simulink model "ExtendedLQR"  (R2020b)
settings: Solver=ode45  StartTime=0.0  StopTime=3  RelTol=1e-4
values from neighbouring files (symbols this model uses):
  degs2rpm = 60/360    (= 0.166666666667)    [load_params_inertial_case.m]
  rads2rpm = 60/2/pi    (= 9.54929658551)    [load_params_inertial_case.m]
  rpm2rads = 2*pi/60    (= 0.10471975512)    [load_params_inertial_case.m]
undefined symbols (not defined in the file or in its folder): daq, drv, extended_bryson_lqr, extended_lqr, gbox, mld, mot, sens, state_space
settings Model: Creator=Utente  LastModifiedBy=Utente
settings SolverCC: ZeroCrossAlgorithm=Adaptive
settings DataIOCC: ReturnWorkspaceOutputs=off
settings DebuggingCC: IgnoredZcDiagnostic=none

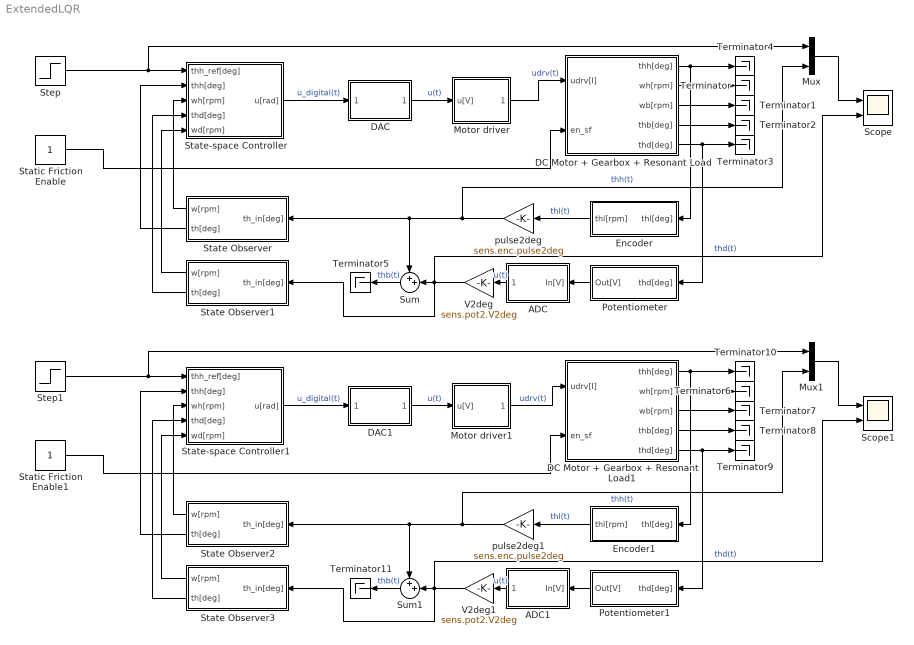
== system ExtendedLQR ==
  ADC : Subsystem
  ADC1 : Subsystem
  DAC : Subsystem
  DAC1 : Subsystem
  DC Motor + Gearbox + Resonant Load : Subsystem
  DC Motor + Gearbox + Resonant Load1 : Subsystem
  Encoder : Subsystem
  Encoder1 : Subsystem
  Motor driver : Subsystem
  Motor driver1 : Subsystem
  Mux : Mux  Inputs=2
  Mux1 : Mux  Inputs=2
  Potentiometer : Subsystem
  Potentiometer1 : Subsystem
  Scope : Scope  NumInputPorts=2
  Scope1 : Scope  NumInputPorts=2
  State Observer : Subsystem
  State Observer1 : Subsystem
  State Observer2 : Subsystem
  State Observer3 : Subsystem
  State-space Controller : Subsystem
  State-space Controller1 : Subsystem
  Static Friction Enable : Constant
  Static Friction Enable1 : Constant
  Step : Step  Time=0  After=50  SampleTime=0
  Step1 : Step  Time=0  After=50  SampleTime=0
  Sum : Sum  Inputs=++|
  Sum1 : Sum  Inputs=++|
  Terminator{,1..11} (12 alike) : Terminator
  V2deg : Gain  Gain=sens.pot2.V2deg
  V2deg1 : Gain  Gain=sens.pot2.V2deg
  pulse2deg : Gain  Gain=sens.enc.pulse2deg
  pulse2deg1 : Gain  Gain=sens.enc.pulse2deg
  wires:
  DC Motor + Gearbox + Resonant Load/5(thd[deg]) -> Terminator3/1, Potentiometer/1(thd[deg])
  DC Motor + Gearbox + Resonant Load/1(thh[deg]) -> Terminator4/1, Encoder/1(thl[deg])
  DC Motor + Gearbox + Resonant Load/2(wh[rpm]) -> Terminator/1
  DC Motor + Gearbox + Resonant Load/3(wb[rpm]) -> Terminator1/1
  DC Motor + Gearbox + Resonant Load/4(thb[deg]) -> Terminator2/1
  Encoder/1(thl[rpm]) -> pulse2deg/1  "thl(t)"
  V2deg/1 -> State Observer1/1(th_in[deg]), Scope/2, Sum/2  "thd(t)"
  pulse2deg/1 -> Mux/2, State Observer/1(th_in[deg]), Sum/1  "thh(t)"
  Motor driver/1(udrv[I]) -> DC Motor + Gearbox + Resonant Load/1(udrv[I])  "udrv(t)"
  DAC/1(Out[V]) -> Motor driver/1(u[V])  "u(t)"
  ADC/1(Out[V]) -> V2deg/1  "u(t)"
  Potentiometer/1(Out[V]) -> ADC/1(In[V])
  State-space Controller/1(u[rad]) -> DAC/1(In[rad])  "u_digital(t)"
  Step/1 -> State-space Controller/1(thh_ref[deg]), Mux/1
  Mux/1 -> Scope/1
  State Observer/1(w[rpm]) -> State-space Controller/3(wh[rpm])
  State Observer/2(th[deg]) -> State-space Controller/2(thh[deg])
  State Observer1/1(w[rpm]) -> State-space Controller/5(wd[rpm])
  State Observer1/2(th[deg]) -> State-space Controller/4(thd[deg])
  Sum/1 -> Terminator5/1  "thb(t)"
  Static Friction Enable/1 -> DC Motor + Gearbox + Resonant Load/2(en_sf)
  Step1/1 -> State-space Controller1/1(thh_ref[deg]), Mux1/1
  Static Friction Enable1/1 -> DC Motor + Gearbox + Resonant Load1/2(en_sf)
  State Observer2/2(th[deg]) -> State-space Controller1/2(thh[deg])
  Potentiometer1/1(Out[V]) -> ADC1/1(In[V])
  State Observer3/1(w[rpm]) -> State-space Controller1/5(wd[rpm])
  State Observer3/2(th[deg]) -> State-space Controller1/4(thd[deg])
  Encoder1/1(thl[rpm]) -> pulse2deg1/1  "thl(t)"
  V2deg1/1 -> State Observer3/1(th_in[deg]), Scope1/2, Sum1/2  "thd(t)"
  DAC1/1(Out[V]) -> Motor driver1/1(u[V])  "u(t)"
  State-space Controller1/1(u[rad]) -> DAC1/1(In[rad])  "u_digital(t)"
  Mux1/1 -> Scope1/1
  State Observer2/1(w[rpm]) -> State-space Controller1/3(wh[rpm])
  DC Motor + Gearbox + Resonant Load1/3(wb[rpm]) -> Terminator7/1
  ADC1/1(Out[V]) -> V2deg1/1  "u(t)"
  DC Motor + Gearbox + Resonant Load1/1(thh[deg]) -> Terminator10/1, Encoder1/1(thl[deg])
  Sum1/1 -> Terminator11/1  "thb(t)"
  Motor driver1/1(udrv[I]) -> DC Motor + Gearbox + Resonant Load1/1(udrv[I])  "udrv(t)"
  DC Motor + Gearbox + Resonant Load1/4(thb[deg]) -> Terminator8/1
  pulse2deg1/1 -> Mux1/2, State Observer2/1(th_in[deg]), Sum1/1  "thh(t)"
  DC Motor + Gearbox + Resonant Load1/2(wh[rpm]) -> Terminator6/1
  DC Motor + Gearbox + Resonant Load1/5(thd[deg]) -> Terminator9/1, Potentiometer1/1(thd[deg])

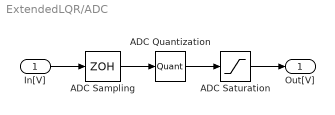
== system ExtendedLQR/ADC ==
  In[V] : Inport
  ADC Quantization : Quantizer  QuantizationInterval=daq.adc.q
  ADC Sampling : ZeroOrderHold  SampleTime=daq.adc.T_s
  ADC Saturation : Saturate  UpperLimit=daq.adc.vdd  LowerLimit=daq.adc.vss
  Out[V] : Outport
  wires:
  ADC Quantization/1 -> ADC Saturation/1
  ADC Sampling/1 -> ADC Quantization/1
  ADC Saturation/1 -> Out[V]/1
  In[V]/1 -> ADC Sampling/1

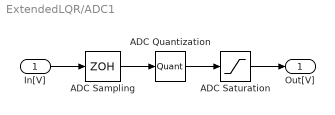
== system ExtendedLQR/ADC1 ==
  In[V] : Inport
  ADC Quantization : Quantizer  QuantizationInterval=daq.adc.q
  ADC Sampling : ZeroOrderHold  SampleTime=daq.adc.T_s
  ADC Saturation : Saturate  UpperLimit=daq.adc.vdd  LowerLimit=daq.adc.vss
  Out[V] : Outport
  wires:
  ADC Quantization/1 -> ADC Saturation/1
  ADC Sampling/1 -> ADC Quantization/1
  ADC Saturation/1 -> Out[V]/1
  In[V]/1 -> ADC Sampling/1

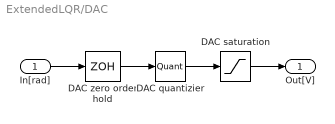
== system ExtendedLQR/DAC ==
  In[rad] : Inport
  DAC quantizier : Quantizer  QuantizationInterval=daq.dac.q
  DAC saturation : Saturate  UpperLimit=daq.dac.vdd  LowerLimit=daq.dac.vss
  DAC zero order hold : ZeroOrderHold  SampleTime=daq.dac.T_s
  Out[V] : Outport
  wires:
  DAC quantizier/1 -> DAC saturation/1
  DAC zero order hold/1 -> DAC quantizier/1
  DAC saturation/1 -> Out[V]/1
  In[rad]/1 -> DAC zero order hold/1

== system ExtendedLQR/DAC1 ==
  In[rad] : Inport
  DAC quantizier : Quantizer  QuantizationInterval=daq.dac.q
  DAC saturation : Saturate  UpperLimit=daq.dac.vdd  LowerLimit=daq.dac.vss
  DAC zero order hold : ZeroOrderHold  SampleTime=daq.dac.T_s
  Out[V] : Outport
  wires:
  DAC quantizier/1 -> DAC saturation/1
  DAC zero order hold/1 -> DAC quantizier/1
  DAC saturation/1 -> Out[V]/1
  In[rad]/1 -> DAC zero order hold/1

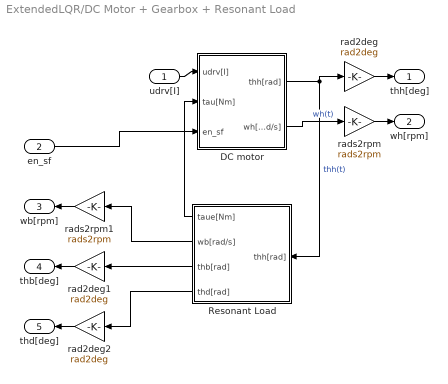
== system ExtendedLQR/DC Motor + Gearbox + Resonant Load ==
  udrv[I] : Inport
  en_sf : Inport  Port=2
  DC motor : Subsystem
  Resonant Load : Subsystem
  rad2deg : Gain  Gain=rad2deg
  rad2deg1 : Gain  Gain=rad2deg
  rad2deg2 : Gain  Gain=rad2deg
  rads2rpm : Gain  Gain=rads2rpm
  rads2rpm1 : Gain  Gain=rads2rpm
  thh[deg] : Outport
  wh[rpm] : Outport  Port=2
  wb[rpm] : Outport  Port=3
  thb[deg] : Outport  Port=4
  thd[deg] : Outport  Port=5
  wires:
  rad2deg2/1 -> thd[deg]/1
  rad2deg1/1 -> thb[deg]/1
  DC motor/1(thh[rad]) -> rad2deg/1, Resonant Load/1(thh[rad])  "thh(t)"
  Resonant Load/2(wb[rad/s]) -> rads2rpm1/1
  Resonant Load/4(thd[rad]) -> rad2deg2/1
  Resonant Load/3(thb[rad]) -> rad2deg1/1
  DC motor/2(wh[rad/s]) -> rads2rpm/1  "wh(t)"
  udrv[I]/1 -> DC motor/1(udrv[I])
  rad2deg/1 -> thh[deg]/1
  rads2rpm/1 -> wh[rpm]/1
  rads2rpm1/1 -> wb[rpm]/1
  Resonant Load/1(taue[Nm]) -> DC motor/2(tau[Nm])
  en_sf/1 -> DC motor/3(en_sf)

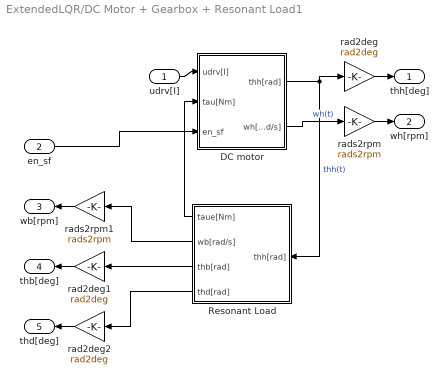
== system ExtendedLQR/DC Motor + Gearbox + Resonant Load1 ==
  udrv[I] : Inport
  en_sf : Inport  Port=2
  DC motor : Subsystem
  Resonant Load : Subsystem
  rad2deg : Gain  Gain=rad2deg
  rad2deg1 : Gain  Gain=rad2deg
  rad2deg2 : Gain  Gain=rad2deg
  rads2rpm : Gain  Gain=rads2rpm
  rads2rpm1 : Gain  Gain=rads2rpm
  thh[deg] : Outport
  wh[rpm] : Outport  Port=2
  wb[rpm] : Outport  Port=3
  thb[deg] : Outport  Port=4
  thd[deg] : Outport  Port=5
  wires:
  rad2deg2/1 -> thd[deg]/1
  rad2deg1/1 -> thb[deg]/1
  DC motor/1(thh[rad]) -> rad2deg/1, Resonant Load/1(thh[rad])  "thh(t)"
  Resonant Load/2(wb[rad/s]) -> rads2rpm1/1
  Resonant Load/4(thd[rad]) -> rad2deg2/1
  Resonant Load/3(thb[rad]) -> rad2deg1/1
  DC motor/2(wh[rad/s]) -> rads2rpm/1  "wh(t)"
  udrv[I]/1 -> DC motor/1(udrv[I])
  rad2deg/1 -> thh[deg]/1
  rads2rpm/1 -> wh[rpm]/1
  rads2rpm1/1 -> wb[rpm]/1
  Resonant Load/1(taue[Nm]) -> DC motor/2(tau[Nm])
  en_sf/1 -> DC motor/3(en_sf)

== system ExtendedLQR/Encoder ==
  thl[deg] : Inport
  Encoder quantization : Quantizer  QuantizationInterval=sens.enc.q
  Encoder sampling : ZeroOrderHold  SampleTime=sens.enc.T_s
  deg2pulse : Gain  Gain=sens.enc.deg2pulse
  thl[rpm] : Outport
  wires:
  Encoder quantization/1 -> deg2pulse/1
  deg2pulse/1 -> thl[rpm]/1
  Encoder sampling/1 -> Encoder quantization/1
  thl[deg]/1 -> Encoder sampling/1

== system ExtendedLQR/Encoder1 ==
  thl[deg] : Inport
  Encoder quantization : Quantizer  QuantizationInterval=sens.enc.q
  Encoder sampling : ZeroOrderHold  SampleTime=sens.enc.T_s
  deg2pulse : Gain  Gain=sens.enc.deg2pulse
  thl[rpm] : Outport
  wires:
  Encoder quantization/1 -> deg2pulse/1
  deg2pulse/1 -> thl[rpm]/1
  Encoder sampling/1 -> Encoder quantization/1
  thl[deg]/1 -> Encoder sampling/1

== system ExtendedLQR/Motor driver ==
  u[V] : Inport
  Driver dynamics : TransferFcn  Numerator=[drv.dcgain]  Denominator=[drv.Tc 1]
  Driver saturation : Saturate  UpperLimit=drv.vp  LowerLimit=drv.vm
  udrv[I] : Outport
  wires:
  Driver saturation/1 -> udrv[I]/1
  Driver dynamics/1 -> Driver saturation/1
  u[V]/1 -> Driver dynamics/1

== system ExtendedLQR/Motor driver1 ==
  u[V] : Inport
  Driver dynamics : TransferFcn  Numerator=[drv.dcgain]  Denominator=[drv.Tc 1]
  Driver saturation : Saturate  UpperLimit=drv.vp  LowerLimit=drv.vm
  udrv[I] : Outport
  wires:
  Driver saturation/1 -> udrv[I]/1
  Driver dynamics/1 -> Driver saturation/1
  u[V]/1 -> Driver dynamics/1

== system ExtendedLQR/Potentiometer ==
  thd[deg] : Inport
  Sensor Output Noise [V] : RandomNumber  Variance=sens.pot2.noise.var  SampleTime=0.1
  Sum : Sum  Inputs=|++
  deg2V : Gain  Gain=sens.pot2.deg2V
  Out[V] : Outport
  wires:
  thd[deg]/1 -> deg2V/1
  Sensor Output Noise [V]/1 -> Sum/2
  deg2V/1 -> Sum/1
  Sum/1 -> Out[V]/1

== system ExtendedLQR/Potentiometer1 ==
  thd[deg] : Inport
  Sensor Output Noise [V] : RandomNumber  Variance=sens.pot2.noise.var  SampleTime=0.1
  Sum : Sum  Inputs=|++
  deg2V : Gain  Gain=sens.pot2.deg2V
  Out[V] : Outport
  wires:
  thd[deg]/1 -> deg2V/1
  Sensor Output Noise [V]/1 -> Sum/2
  deg2V/1 -> Sum/1
  Sum/1 -> Out[V]/1

== system ExtendedLQR/State Observer ==
  th_in[deg] : Inport
  Derivator : TransferFcn  Numerator=[state_space.obs.wc^2 0]  Denominator=[1 2*state_space.obs.delta*state_space.obs.wc state_space.obs.wc^2]
  degs2rpm : Gain  Gain=degs2rpm
  w[rpm] : Outport
  th[deg] : Outport  Port=2
  wires:
  Derivator/1 -> degs2rpm/1
  th_in[deg]/1 -> th[deg]/1, Derivator/1
  degs2rpm/1 -> w[rpm]/1

== system ExtendedLQR/State Observer1 ==
  th_in[deg] : Inport
  Transfer Fcn : TransferFcn  Numerator=[state_space.obs.wc^2 0]  Denominator=[1 2*state_space.obs.delta*state_space.obs.wc state_space.obs.wc^2]
  degs2rpm : Gain  Gain=degs2rpm
  w[rpm] : Outport
  th[deg] : Outport  Port=2
  wires:
  Transfer Fcn/1 -> degs2rpm/1
  th_in[deg]/1 -> th[deg]/1, Transfer Fcn/1
  degs2rpm/1 -> w[rpm]/1

== system ExtendedLQR/State Observer2 ==
  th_in[deg] : Inport
  Derivator : TransferFcn  Numerator=[state_space.obs.wc^2 0]  Denominator=[1 2*state_space.obs.delta*state_space.obs.wc state_space.obs.wc^2]
  degs2rpm : Gain  Gain=degs2rpm
  w[rpm] : Outport
  th[deg] : Outport  Port=2
  wires:
  Derivator/1 -> degs2rpm/1
  th_in[deg]/1 -> th[deg]/1, Derivator/1
  degs2rpm/1 -> w[rpm]/1

== system ExtendedLQR/State Observer3 ==
  th_in[deg] : Inport
  Transfer Fcn : TransferFcn  Numerator=[state_space.obs.wc^2 0]  Denominator=[1 2*state_space.obs.delta*state_space.obs.wc state_space.obs.wc^2]
  degs2rpm : Gain  Gain=degs2rpm
  w[rpm] : Outport
  th[deg] : Outport  Port=2
  wires:
  Transfer Fcn/1 -> degs2rpm/1
  th_in[deg]/1 -> th[deg]/1, Transfer Fcn/1
  degs2rpm/1 -> w[rpm]/1

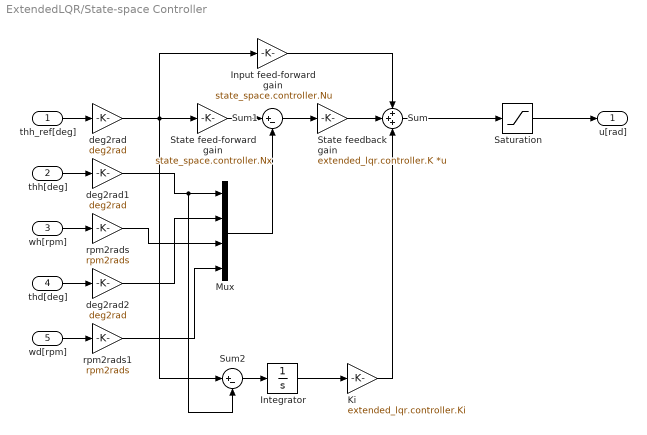
== system ExtendedLQR/State-space Controller ==
  thh_ref[deg] : Inport
  thh[deg] : Inport  Port=2
  wh[rpm] : Inport  Port=3
  thd[deg] : Inport  Port=4
  wd[rpm] : Inport  Port=5
  Input feed-forward gain : Gain  Gain=state_space.controller.Nu
  Integrator : Integrator
  Ki : Gain  Gain=extended_lqr.controller.Ki
  Mux : Mux
  Saturation : Saturate  UpperLimit=daq.dac.vdd  LowerLimit=daq.dac.vss
  State feed-forward gain : Gain  Gain=state_space.controller.Nx
  State feedback gain : Gain  Gain=extended_lqr.controller.K  Multiplication=Matrix(K*u)
  Sum : Sum  Inputs=+++
  Sum1 : Sum  Inputs=|+-
  Sum2 : Sum  Inputs=|+-
  deg2rad : Gain  Gain=deg2rad
  deg2rad1 : Gain  Gain=deg2rad
  deg2rad2 : Gain  Gain=deg2rad
  rpm2rads : Gain  Gain=rpm2rads
  rpm2rads1 : Gain  Gain=rpm2rads
  u[rad] : Outport
  wires:
  Sum1/1 -> State feedback gain/1
  Mux/1 -> Sum1/2
  thh_ref[deg]/1 -> deg2rad/1
  deg2rad/1 -> Sum2/1, Input feed-forward gain/1, State feed-forward gain/1
  State feed-forward gain/1 -> Sum1/1
  Input feed-forward gain/1 -> Sum/1
  Saturation/1 -> u[rad]/1
  wh[rpm]/1 -> rpm2rads/1
  thh[deg]/1 -> deg2rad1/1
  State feedback gain/1 -> Sum/2
  Sum/1 -> Saturation/1
  thd[deg]/1 -> deg2rad2/1
  wd[rpm]/1 -> rpm2rads1/1
  deg2rad1/1 -> Sum2/2, Mux/1
  deg2rad2/1 -> Mux/2
  rpm2rads/1 -> Mux/3
  rpm2rads1/1 -> Mux/4
  Integrator/1 -> Ki/1
  Sum2/1 -> Integrator/1
  Ki/1 -> Sum/3

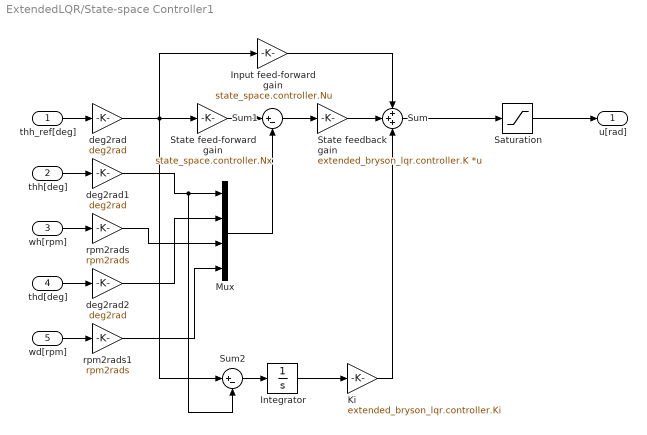
== system ExtendedLQR/State-space Controller1 ==
  thh_ref[deg] : Inport
  thh[deg] : Inport  Port=2
  wh[rpm] : Inport  Port=3
  thd[deg] : Inport  Port=4
  wd[rpm] : Inport  Port=5
  Input feed-forward gain : Gain  Gain=state_space.controller.Nu
  Integrator : Integrator
  Ki : Gain  Gain=extended_bryson_lqr.controller.Ki
  Mux : Mux
  Saturation : Saturate  UpperLimit=daq.dac.vdd  LowerLimit=daq.dac.vss
  State feed-forward gain : Gain  Gain=state_space.controller.Nx
  State feedback gain : Gain  Gain=extended_bryson_lqr.controller.K  Multiplication=Matrix(K*u)
  Sum : Sum  Inputs=+++
  Sum1 : Sum  Inputs=|+-
  Sum2 : Sum  Inputs=|+-
  deg2rad : Gain  Gain=deg2rad
  deg2rad1 : Gain  Gain=deg2rad
  deg2rad2 : Gain  Gain=deg2rad
  rpm2rads : Gain  Gain=rpm2rads
  rpm2rads1 : Gain  Gain=rpm2rads
  u[rad] : Outport
  wires:
  Sum1/1 -> State feedback gain/1
  Mux/1 -> Sum1/2
  thh_ref[deg]/1 -> deg2rad/1
  deg2rad/1 -> Sum2/1, Input feed-forward gain/1, State feed-forward gain/1
  State feed-forward gain/1 -> Sum1/1
  Input feed-forward gain/1 -> Sum/1
  Saturation/1 -> u[rad]/1
  wh[rpm]/1 -> rpm2rads/1
  thh[deg]/1 -> deg2rad1/1
  State feedback gain/1 -> Sum/2
  Sum/1 -> Saturation/1
  thd[deg]/1 -> deg2rad2/1
  wd[rpm]/1 -> rpm2rads1/1
  deg2rad1/1 -> Sum2/2, Mux/1
  deg2rad2/1 -> Mux/2
  rpm2rads/1 -> Mux/3
  rpm2rads1/1 -> Mux/4
  Integrator/1 -> Ki/1
  Sum2/1 -> Integrator/1
  Ki/1 -> Sum/3

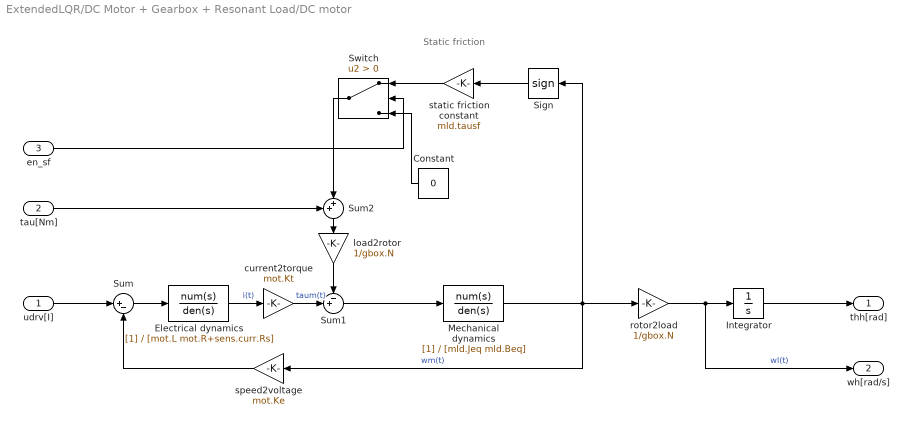
== system ExtendedLQR/DC Motor + Gearbox + Resonant Load/DC motor ==
  note: Static friction
  udrv[I] : Inport  Unit=V
  tau[Nm] : Inport  Port=2  Unit=V
  en_sf : Inport  Port=3  Unit=V
  Constant : Constant  Value=0
  Electrical dynamics : TransferFcn  Denominator=[mot.L mot.R+sens.curr.Rs]
  Integrator : Integrator
  Mechanical dynamics : TransferFcn  Denominator=[mld.Jeq mld.Beq]
  Sign : Signum  ZeroCross=off
  Sum : Sum  Inputs=|+-
  Sum1 : Sum  Inputs=-+|
  Sum2 : Sum  Inputs=++|
  Switch : Switch  Criteria=u2 > Threshold
  current2torque : Gain  Gain=mot.Kt
  load2rotor : Gain  Gain=1/gbox.N
  rotor2load : Gain  Gain=1/gbox.N
  speed2voltage : Gain  Gain=mot.Ke
  static friction constant : Gain  Gain=mld.tausf
  thh[rad] : Outport  Unit=deg
  wh[rad/s] : Outport  Port=2  Unit=rpm
  wires:
  load2rotor/1 -> Sum1/1
  Mechanical dynamics/1 -> Sign/1, rotor2load/1, speed2voltage/1  "wm(t)"
  Sign/1 -> static friction constant/1
  current2torque/1 -> Sum1/2  "taum(t)"
  Sum1/1 -> Mechanical dynamics/1
  speed2voltage/1 -> Sum/2
  rotor2load/1 -> wh[rad/s]/1, Integrator/1  "wl(t)"
  Electrical dynamics/1 -> current2torque/1  "i(t)"
  Sum/1 -> Electrical dynamics/1
  Integrator/1 -> thh[rad]/1
  udrv[I]/1 -> Sum/1
  Sum2/1 -> load2rotor/1
  tau[Nm]/1 -> Sum2/1
  static friction constant/1 -> Switch/1
  Switch/1 -> Sum2/2
  en_sf/1 -> Switch/2
  Constant/1 -> Switch/3

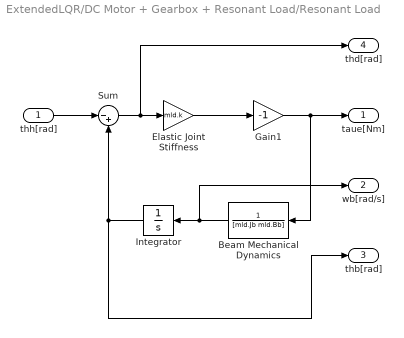
== system ExtendedLQR/DC Motor + Gearbox + Resonant Load/Resonant Load ==
  thh[rad] : Inport
  Beam Mechanical Dynamics : TransferFcn  Denominator=[mld.Jb mld.Bb]
  Elastic Joint Stiffness : Gain  Gain=mld.k
  Gain1 : Gain  Gain=-1
  Integrator : Integrator
  Sum : Sum  Inputs=|-+
  taue[Nm] : Outport
  wb[rad/s] : Outport  Port=2
  thb[rad] : Outport  Port=3
  thd[rad] : Outport  Port=4
  wires:
  Beam Mechanical Dynamics/1 -> wb[rad/s]/1, Integrator/1
  Elastic Joint Stiffness/1 -> Gain1/1
  Gain1/1 -> taue[Nm]/1, Beam Mechanical Dynamics/1
  thh[rad]/1 -> Sum/1
  Integrator/1 -> thb[rad]/1, Sum/2
  Sum/1 -> thd[rad]/1, Elastic Joint Stiffness/1

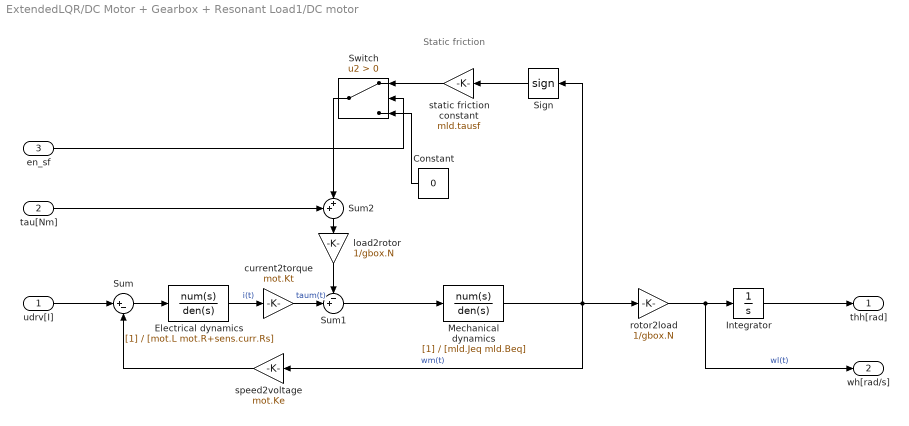
== system ExtendedLQR/DC Motor + Gearbox + Resonant Load1/DC motor ==
  note: Static friction
  udrv[I] : Inport  Unit=V
  tau[Nm] : Inport  Port=2  Unit=V
  en_sf : Inport  Port=3  Unit=V
  Constant : Constant  Value=0
  Electrical dynamics : TransferFcn  Denominator=[mot.L mot.R+sens.curr.Rs]
  Integrator : Integrator
  Mechanical dynamics : TransferFcn  Denominator=[mld.Jeq mld.Beq]
  Sign : Signum  ZeroCross=off
  Sum : Sum  Inputs=|+-
  Sum1 : Sum  Inputs=-+|
  Sum2 : Sum  Inputs=++|
  Switch : Switch  Criteria=u2 > Threshold
  current2torque : Gain  Gain=mot.Kt
  load2rotor : Gain  Gain=1/gbox.N
  rotor2load : Gain  Gain=1/gbox.N
  speed2voltage : Gain  Gain=mot.Ke
  static friction constant : Gain  Gain=mld.tausf
  thh[rad] : Outport  Unit=deg
  wh[rad/s] : Outport  Port=2  Unit=rpm
  wires:
  load2rotor/1 -> Sum1/1
  Mechanical dynamics/1 -> Sign/1, rotor2load/1, speed2voltage/1  "wm(t)"
  Sign/1 -> static friction constant/1
  current2torque/1 -> Sum1/2  "taum(t)"
  Sum1/1 -> Mechanical dynamics/1
  speed2voltage/1 -> Sum/2
  rotor2load/1 -> wh[rad/s]/1, Integrator/1  "wl(t)"
  Electrical dynamics/1 -> current2torque/1  "i(t)"
  Sum/1 -> Electrical dynamics/1
  Integrator/1 -> thh[rad]/1
  udrv[I]/1 -> Sum/1
  Sum2/1 -> load2rotor/1
  tau[Nm]/1 -> Sum2/1
  static friction constant/1 -> Switch/1
  Switch/1 -> Sum2/2
  en_sf/1 -> Switch/2
  Constant/1 -> Switch/3

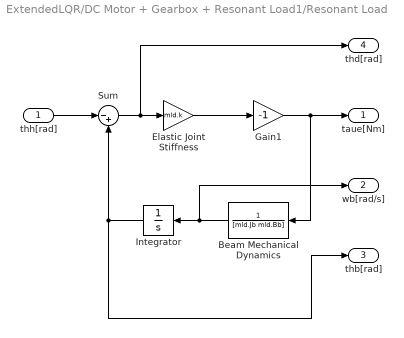
== system ExtendedLQR/DC Motor + Gearbox + Resonant Load1/Resonant Load ==
  thh[rad] : Inport
  Beam Mechanical Dynamics : TransferFcn  Denominator=[mld.Jb mld.Bb]
  Elastic Joint Stiffness : Gain  Gain=mld.k
  Gain1 : Gain  Gain=-1
  Integrator : Integrator
  Sum : Sum  Inputs=|-+
  taue[Nm] : Outport
  wb[rad/s] : Outport  Port=2
  thb[rad] : Outport  Port=3
  thd[rad] : Outport  Port=4
  wires:
  Beam Mechanical Dynamics/1 -> wb[rad/s]/1, Integrator/1
  Elastic Joint Stiffness/1 -> Gain1/1
  Gain1/1 -> taue[Nm]/1, Beam Mechanical Dynamics/1
  thh[rad]/1 -> Sum/1
  Integrator/1 -> thb[rad]/1, Sum/2
  Sum/1 -> thd[rad]/1, Elastic Joint Stiffness/1
